simulink model "Realizacoes_Simulink_2015b"  (R2015b)
settings: Solver=ode45  SolverMode=SingleTasking  StartTime=0.0  StopTime=10.0  RelTol=1e-3
libraries: dsparch4 x4
settings Model: Creator=marco  LastModifiedBy=marco
settings DataIOCC: LimitDataPoints=off
settings DebuggingCC: AllowSymbolicDim=on  SFUnexpectedBacktrackingDiag=error  SFNoUnconditionalDefaultTransitionDiag=error
settings HardwareCC: ProdWordSize=32  ProdHWDeviceType=Specified
settings ModelReferenceCC: PropagateSignalLabelsOutOfModel=on
settings GRTTargetCC: TargetLangStandard=C99 (ISO)
settings ConfigComp: CovMetricSettings=dwe  CovHtmlReporting=off  CovSaveCumulativeToWorkspaceVar=off  CovSaveSingleToWorkspaceVar=off  CovModelRefEnable=Off  CovExternalEMLEnable=on

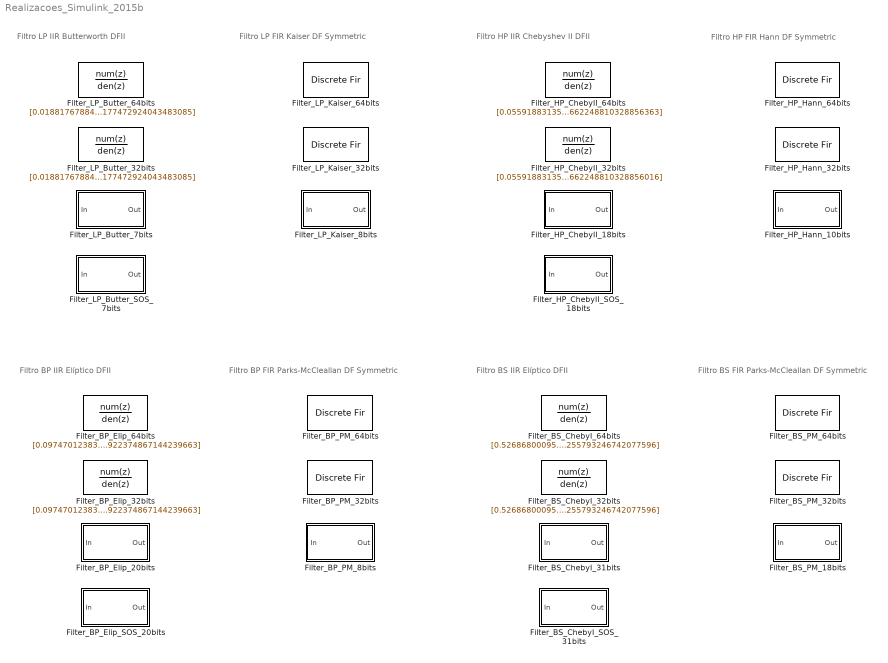
== system Realizacoes_Simulink_2015b ==
  note: Filtro LP IIR Butterworth DFII
  note: Filtro LP FIR Kaiser DF Symmetric
  note: Filtro HP IIR Chebyshev II DFII
  note: Filtro HP FIR Hann DF Symmetric
  note: Filtro BP IIR Elíptico DFII
  note: Filtro BP FIR Parks-McCleallan DF Symmetric
  note: Filtro BS IIR Elíptico DFII
  note: Filtro BS FIR Parks-McCleallan DF Symmetric
  Filter_BP_Elip_20bits : Subsystem  Tag=BlockMethodSubSystem
  Filter_BP_Elip_32bits : DiscreteFilter  Tag=BlockMethodSubSystem  Numerator=[0.0974701238336903308 0.132939383916824333 0.234899653984624923 0.132939383916824333 0.0974701238336903308]  Denominator=[1 1.35628195146766672 2.3760241493758163 1.30250572686881982 0.922374867144239663]  InputProcessing=Columns as channels (frame based)  a0EqualsOne=on
  Filter_BP_Elip_64bits : DiscreteFilter  Tag=BlockMethodSubSystem  Numerator=[0.0974701238336903308 0.132939383916824333 0.234899653984624923 0.132939383916824333 0.0974701238336903308]  Denominator=[1 1.35628195146766672 2.3760241493758163 1.30250572686881982 0.922374867144239663]  InputProcessing=Columns as channels (frame based)  a0EqualsOne=on
  Filter_BP_Elip_SOS_20bits : Subsystem  Tag=BlockMethodSubSystem
  Filter_BP_PM_32bits : DiscreteFir  Tag=BlockMethodSubSystem  FilterStructure=Direct form symmetric  Coefficients=[-0.0433412092937293658 0.00428125381265335829 0.00433549487836447974 0.00392877576103001919 0.00473672650552339151 -0.00113536747739367079 0.00225664087871407099 0.0129845358018076552 -0.00161672199950467889 -0.0104604010793571591 0.0163185558804867653 0.0128200383399435375 -0.0195811015916752505 0.00139459356195246087 0.0265908628917521095 -0.00801815848233358545 -0.0159846853288865345 0.0182879102661886624 0.00917068699111520461 -0.0101571946073742616 0.00213367932078208566 0.00146979326149086938 0.00584552068680904268 0.0142736412678231232 -0.0203435807946345457 -0.0109359709753772891 0.0481729986576425739 -0.00509592495312094235 -0.0617262707720767426 0.0445756327859687662 0.0603830661005346145 -0.0814319206649492117 -0.026284446547936522 0.110018542760450824 -0.0206200310747097909 -0.10438558333404982 0.0746608800226218894 0.0746608800226218894 -0.10438558333404982 -0.0206200310747097909 0.110018542760450824 -0.026284446547936522 -0.0814319206649492117 0.0603830661005346145 0.0445756327859687662 -0.0617262707720767426 -0.00509592495312094235 0.0481729986576425739 -0.0109359709753772891 -0.0203435807946345457 0.0142736412678231232 0.00584552068680904268 0.00146979326149086938 0.00213367932078208566 -0.0101571946073742616 0.00917068699111520461 0.0182879102661886624 -0.0159846853288865345 -0.00801815848233358545 0.0265908628917521095 0.00139459356195246087 -0.0195811015916752505 0.0128200383399435375 0.0163185558804867653 -0.0104604010793571591 -0.00161672199950467889 0.0129845358018076552 0.00225664087871407099 -0.00113536747739367079 0.00473672650552339151 0.00392877576103001919 0.00433549487836447974 0.00428125381265335829 -0.0433412092937293658]  InputProcessing=Columns as channels (frame based)
  Filter_BP_PM_64bits : DiscreteFir  Tag=BlockMethodSubSystem  FilterStructure=Direct form symmetric  Coefficients=[-0.0433412092937293658 0.00428125381265335829 0.00433549487836447974 0.00392877576103001919 0.00473672650552339151 -0.00113536747739367079 0.00225664087871407099 0.0129845358018076552 -0.00161672199950467889 -0.0104604010793571591 0.0163185558804867653 0.0128200383399435375 -0.0195811015916752505 0.00139459356195246087 0.0265908628917521095 -0.00801815848233358545 -0.0159846853288865345 0.0182879102661886624 0.00917068699111520461 -0.0101571946073742616 0.00213367932078208566 0.00146979326149086938 0.00584552068680904268 0.0142736412678231232 -0.0203435807946345457 -0.0109359709753772891 0.0481729986576425739 -0.00509592495312094235 -0.0617262707720767426 0.0445756327859687662 0.0603830661005346145 -0.0814319206649492117 -0.026284446547936522 0.110018542760450824 -0.0206200310747097909 -0.10438558333404982 0.0746608800226218894 0.0746608800226218894 -0.10438558333404982 -0.0206200310747097909 0.110018542760450824 -0.026284446547936522 -0.0814319206649492117 0.0603830661005346145 0.0445756327859687662 -0.0617262707720767426 -0.00509592495312094235 0.0481729986576425739 -0.0109359709753772891 -0.0203435807946345457 0.0142736412678231232 0.00584552068680904268 0.00146979326149086938 0.00213367932078208566 -0.0101571946073742616 0.00917068699111520461 0.0182879102661886624 -0.0159846853288865345 -0.00801815848233358545 0.0265908628917521095 0.00139459356195246087 -0.0195811015916752505 0.0128200383399435375 0.0163185558804867653 -0.0104604010793571591 -0.00161672199950467889 0.0129845358018076552 0.00225664087871407099 -0.00113536747739367079 0.00473672650552339151 0.00392877576103001919 0.00433549487836447974 0.00428125381265335829 -0.0433412092937293658]  InputProcessing=Columns as channels (frame based)
  Filter_BP_PM_8bits : Subsystem  Tag=BlockMethodSubSystem
  Filter_BS_ChebyI_31bits : Subsystem  Tag=BlockMethodSubSystem
  Filter_BS_ChebyI_32bits : DiscreteFilter  Tag=BlockMethodSubSystem  Numerator=[0.526868000951233872 -1.54203566956132732 5.62231543277647106 -10.600101182726668 21.298995446777635 -28.6634656336700679 39.4931897641130405 -39.2119772064789842 39.4931897641130405 -28.6634656336700679 21.298995446777635 -10.600101182726668 5.62231543277647106 -1.54203566956132732 0.526868000951233872]  Denominator=[1 -2.66499543662062877 8.79464618040259083 -15.0964799784515531 27.5316314023528577 -33.7583267920149481 42.2783703159670097 -38.2580281440592245 35.0287520822531278 -23.1519310706400248 15.6125822995039183 -7.05648534288835538 3.38096176201517462 -0.836935413720374832 0.255793246742077596]  InputProcessing=Columns as channels (frame based)  a0EqualsOne=on
  Filter_BS_ChebyI_64bits : DiscreteFilter  Tag=BlockMethodSubSystem  Numerator=[0.526868000951233872 -1.54203566956132732 5.62231543277647106 -10.600101182726668 21.298995446777635 -28.6634656336700679 39.4931897641130405 -39.2119772064789842 39.4931897641130405 -28.6634656336700679 21.298995446777635 -10.600101182726668 5.62231543277647106 -1.54203566956132732 0.526868000951233872]  Denominator=[1 -2.66499543662062877 8.79464618040259083 -15.0964799784515531 27.5316314023528577 -33.7583267920149481 42.2783703159670097 -38.2580281440592245 35.0287520822531278 -23.1519310706400248 15.6125822995039183 -7.05648534288835538 3.38096176201517462 -0.836935413720374832 0.255793246742077596]  InputProcessing=Columns as channels (frame based)  a0EqualsOne=on
  Filter_BS_ChebyI_SOS_31bits : Subsystem  Tag=BlockMethodSubSystem
  Filter_BS_PM_18bits : Subsystem  Tag=BlockMethodSubSystem
  Filter_BS_PM_32bits : DiscreteFir  Tag=BlockMethodSubSystem  FilterStructure=Direct form symmetric  Coefficients=[0.00939244855741547431 0.00168644324503250398 -0.00123334499269933651 0.00145794752474150894 -0.00170828863653412779 0.0010371674316927424 -0.000634686404143752943 0.00136311298569206278 -0.00129284830014917774 0.000232789421018792837 -0.000621585322147632049 0.00144095326498087451 -0.000402030343464907663 -9.93042424858531166e-05 -0.00117660388067255444 0.000857139817899975971 0.000475576697520832179 0.000566173937320908283 -0.00129976912049715575 -0.000414918760660079426 0.000263301821986200587 0.00151212084328995505 -0.000171353338375926384 -0.00112518747007188781 -0.00113282518202952216 0.00125058626817034176 0.00146260931159716097 -0.00012619100443286255 -0.00218391988276047354 -0.000599163053077525877 0.00175579742678911438 0.00189080421318403406 -0.00128579243659506307 -0.00239772150607349757 -4.34676465038889596e-05 0.0027290015939102491 0.00110819243107837312 -0.00210222575652082655 -0.00225246351867029087 0.0012254746073580233 0.00261463097525626523 0.000119119214611603793 -0.00253564082558753109 -0.00111637470738218088 0.00170231695003329351 0.0017923627508501939 -0.000727566262942802317 -0.00168402489413071446 -0.000261006656951355608 0.00111369062092454233 0.000654612245855574885 -0.000158605418687098992 -0.000457463191175657845 -0.000559561716121999351 -0.000429555092511704057 0.000760465989380783021 0.00154704577781028811 -8.44810420930140716e-05 -0.00249135328445494394 -0.00131792635448624794 0.00265371689363126401 0.00316577013999892612 -0.00178383712812358436 -0.00478209301742398528 -0.000189000463802546241 0.00558218019101575438 0.00283295693765036683 -0.00504693179469161649 -0.00550420058891909654 0.00310083210861084209 0.00739810128662848118 -3.7561071877213364e-05 -0.00788788074996699812 -0.00340775056067187066 0.00667687326885402742 0.00636929503958767306 -0.00400990072987689964 -0.00801845006079115671 0.00053623232732529229 0.00794278817684213219 0.00277147287738032603 -0.00620795501729334842 -0.00501710520110652813 0.00345225121082729913 0.00561809289207314613 -0.000643298312946369495 -0.0045743241567087296 -0.00120667662953364099 0.00248497965148512584 0.00142397294255552594 -0.000397370928880265591 5.34429434601102151e-05 -0.00054191978616790191 -0.00257813916748243126 -0.000500070247838573585 0.00493849669387566321 0.00366520397101527135 -0.00570692659790642421 -0.00825547169902910057 0.00374480093323882818 0.0128097446690955755 0.00134623112172494548 -0.0154780089784019269 -0.00894575142573483979 0.0145725727441816961 0.0174015202645732385 -0.00914885091284967263 -0.0243958071824043887 -0.000547986162959933723 0.0275080274094623607 0.012973139792518764 -0.0249501799896123012 -0.0254965656220924528 0.0161544829725067465 0.0350081953796367931 -0.00211835663899300006 -0.0387033973848105659 -0.0146670495089108472 0.0348621258612269377 0.030722101647759549 -0.023428042785332507 -0.0423658434161012024 0.00615888494345044873 0.0466417749018884706 0.0136734482850623812 -0.042103679691225207 -0.0319882017787958411 0.0292412271592478595 0.0448778449051016048 -0.0104622924834579488 0.922115113062917713 -0.0104622924834579488 0.0448778449051016048 0.0292412271592478595 -0.0319882017787958411 -0.042103679691225207 0.0136734482850623812 0.0466417749018884706 0.00615888494345044873 -0.0423658434161012024 -0.023428042785332507 0.030722101647759549 0.0348621258612269377 -0.0146670495089108472 -0.0387033973848105659 -0.00211835663899300006 0.0350081953796367931 0.0161544829725067465 -0.0254965656220924528 -0.0249501799896123012 0.012973139792518764 0.0275080274094623607 -0.000547986162959933723 -0.0243958071824043887 -0.00914885091284967263 0.0174015202645732385 0.0145725727441816961 -0.00894575142573483979 -0.0154780089784019269 0.00134623112172494548 0.0128097446690955755 0.00374480093323882818 -0.00825547169902910057 -0.00570692659790642421 0.00366520397101527135 0.00493849669387566321 -0.000500070247838573585 -0.00257813916748243126 -0.00054191978616790191 5.34429434601102151e-05 -0.000397370928880265591 ...(+2138 chars)]  InputProcessing=Columns as channels (frame based)
  Filter_BS_PM_64bits : DiscreteFir  Tag=BlockMethodSubSystem  FilterStructure=Direct form symmetric  Coefficients=[0.00939244855741547431 0.00168644324503250398 -0.00123334499269933651 0.00145794752474150894 -0.00170828863653412779 0.0010371674316927424 -0.000634686404143752943 0.00136311298569206278 -0.00129284830014917774 0.000232789421018792837 -0.000621585322147632049 0.00144095326498087451 -0.000402030343464907663 -9.93042424858531166e-05 -0.00117660388067255444 0.000857139817899975971 0.000475576697520832179 0.000566173937320908283 -0.00129976912049715575 -0.000414918760660079426 0.000263301821986200587 0.00151212084328995505 -0.000171353338375926384 -0.00112518747007188781 -0.00113282518202952216 0.00125058626817034176 0.00146260931159716097 -0.00012619100443286255 -0.00218391988276047354 -0.000599163053077525877 0.00175579742678911438 0.00189080421318403406 -0.00128579243659506307 -0.00239772150607349757 -4.34676465038889596e-05 0.0027290015939102491 0.00110819243107837312 -0.00210222575652082655 -0.00225246351867029087 0.0012254746073580233 0.00261463097525626523 0.000119119214611603793 -0.00253564082558753109 -0.00111637470738218088 0.00170231695003329351 0.0017923627508501939 -0.000727566262942802317 -0.00168402489413071446 -0.000261006656951355608 0.00111369062092454233 0.000654612245855574885 -0.000158605418687098992 -0.000457463191175657845 -0.000559561716121999351 -0.000429555092511704057 0.000760465989380783021 0.00154704577781028811 -8.44810420930140716e-05 -0.00249135328445494394 -0.00131792635448624794 0.00265371689363126401 0.00316577013999892612 -0.00178383712812358436 -0.00478209301742398528 -0.000189000463802546241 0.00558218019101575438 0.00283295693765036683 -0.00504693179469161649 -0.00550420058891909654 0.00310083210861084209 0.00739810128662848118 -3.7561071877213364e-05 -0.00788788074996699812 -0.00340775056067187066 0.00667687326885402742 0.00636929503958767306 -0.00400990072987689964 -0.00801845006079115671 0.00053623232732529229 0.00794278817684213219 0.00277147287738032603 -0.00620795501729334842 -0.00501710520110652813 0.00345225121082729913 0.00561809289207314613 -0.000643298312946369495 -0.0045743241567087296 -0.00120667662953364099 0.00248497965148512584 0.00142397294255552594 -0.000397370928880265591 5.34429434601102151e-05 -0.00054191978616790191 -0.00257813916748243126 -0.000500070247838573585 0.00493849669387566321 0.00366520397101527135 -0.00570692659790642421 -0.00825547169902910057 0.00374480093323882818 0.0128097446690955755 0.00134623112172494548 -0.0154780089784019269 -0.00894575142573483979 0.0145725727441816961 0.0174015202645732385 -0.00914885091284967263 -0.0243958071824043887 -0.000547986162959933723 0.0275080274094623607 0.012973139792518764 -0.0249501799896123012 -0.0254965656220924528 0.0161544829725067465 0.0350081953796367931 -0.00211835663899300006 -0.0387033973848105659 -0.0146670495089108472 0.0348621258612269377 0.030722101647759549 -0.023428042785332507 -0.0423658434161012024 0.00615888494345044873 0.0466417749018884706 0.0136734482850623812 -0.042103679691225207 -0.0319882017787958411 0.0292412271592478595 0.0448778449051016048 -0.0104622924834579488 0.922115113062917713 -0.0104622924834579488 0.0448778449051016048 0.0292412271592478595 -0.0319882017787958411 -0.042103679691225207 0.0136734482850623812 0.0466417749018884706 0.00615888494345044873 -0.0423658434161012024 -0.023428042785332507 0.030722101647759549 0.0348621258612269377 -0.0146670495089108472 -0.0387033973848105659 -0.00211835663899300006 0.0350081953796367931 0.0161544829725067465 -0.0254965656220924528 -0.0249501799896123012 0.012973139792518764 0.0275080274094623607 -0.000547986162959933723 -0.0243958071824043887 -0.00914885091284967263 0.0174015202645732385 0.0145725727441816961 -0.00894575142573483979 -0.0154780089784019269 0.00134623112172494548 0.0128097446690955755 0.00374480093323882818 -0.00825547169902910057 -0.00570692659790642421 0.00366520397101527135 0.00493849669387566321 -0.000500070247838573585 -0.00257813916748243126 -0.00054191978616790191 5.34429434601102151e-05 -0.000397370928880265591 ...(+2138 chars)]  InputProcessing=Columns as channels (frame based)
  Filter_HP_ChebyII_18bits : Subsystem  Tag=BlockMethodSubSystem
  Filter_HP_ChebyII_32bits : DiscreteFilter  Tag=BlockMethodSubSystem  Numerator=[0.0559188313546608654 -0.136376837541798468 0.237261208219189834 -0.275765557755878132 0.237261208219190084 -0.136376837541798718 0.0559188313546609347]  Denominator=[1 0.877081919298363322 1.20330623409765192 0.426634402615273078 0.249553249203958549 0.0208863375040826173 0.00662248810328856016]  InputProcessing=Columns as channels (frame based)  a0EqualsOne=on
  Filter_HP_ChebyII_64bits : DiscreteFilter  Tag=BlockMethodSubSystem  Numerator=[0.0559188313546608654 -0.13637683754179869 0.237261208219190139 -0.27576555775587841 0.237261208219190139 -0.13637683754179869 0.0559188313546608584]  Denominator=[1 0.877081919298363322 1.20330623409765192 0.426634402615272967 0.249553249203958494 0.0208863375040825895 0.00662248810328856363]  InputProcessing=Columns as channels (frame based)  a0EqualsOne=on
  Filter_HP_ChebyII_SOS_18bits : Subsystem  Tag=BlockMethodSubSystem
  Filter_HP_Hann_10bits : Subsystem  Tag=BlockMethodSubSystem
  Filter_HP_Hann_32bits : DiscreteFir  Tag=BlockMethodSubSystem  FilterStructure=Direct form symmetric  Coefficients=[-3.16228700308905018e-05 6.58621006149563763e-05 0.000776097424594572832 -0.00123190726621532883 -0.00166048429484726384 0.00472150775562455317 0.000207579074215400968 -0.0098865670153832335 0.00661569202063748852 0.013228130452963581 -0.0204947917682235907 -0.00852732671830981441 0.0401741168966580214 -0.0129883671048673984 -0.0612137762552903905 0.0693172305105436287 0.0774510719237060941 -0.303130389651806942 0.413280930834306504 -0.303130389651806942 0.0774510719237060941 0.0693172305105436287 -0.0612137762552903905 -0.0129883671048673984 0.0401741168966580214 -0.00852732671830981441 -0.0204947917682235907 0.013228130452963581 0.00661569202063748852 -0.0098865670153832335 0.000207579074215400968 0.00472150775562455317 -0.00166048429484726384 -0.00123190726621532883 0.000776097424594572832 6.58621006149563763e-05 -3.16228700308905018e-05]  InputProcessing=Columns as channels (frame based)
  Filter_HP_Hann_64bits : DiscreteFir  Tag=BlockMethodSubSystem  FilterStructure=Direct form symmetric  Coefficients=[-3.16228700308905018e-05 6.58621006149563763e-05 0.000776097424594572832 -0.00123190726621532883 -0.00166048429484726384 0.00472150775562455317 0.000207579074215400968 -0.0098865670153832335 0.00661569202063748852 0.013228130452963581 -0.0204947917682235907 -0.00852732671830981441 0.0401741168966580214 -0.0129883671048673984 -0.0612137762552903905 0.0693172305105436287 0.0774510719237060941 -0.303130389651806942 0.413280930834306504 -0.303130389651806942 0.0774510719237060941 0.0693172305105436287 -0.0612137762552903905 -0.0129883671048673984 0.0401741168966580214 -0.00852732671830981441 -0.0204947917682235907 0.013228130452963581 0.00661569202063748852 -0.0098865670153832335 0.000207579074215400968 0.00472150775562455317 -0.00166048429484726384 -0.00123190726621532883 0.000776097424594572832 6.58621006149563763e-05 -3.16228700308905018e-05]  InputProcessing=Columns as channels (frame based)
  Filter_LP_Butter_32bits : DiscreteFilter  Tag=BlockMethodSubSystem  Numerator=[0.0188176788491913188 0.150541430793530551 0.526895007777356872 1.05379001555471374 1.31723751944339229 1.05379001555471374 0.526895007777356872 0.150541430793530551 0.0188176788491913188]  Denominator=[1 0.169613480636834985 1.0725472360938022 0.126588905837326127 0.296672196811545885 0.0216830884738356162 0.0209853628033078755 0.000713622450830073379 0.000177472924043483085]  InputProcessing=Columns as channels (frame based)  a0EqualsOne=on
  Filter_LP_Butter_64bits : DiscreteFilter  Tag=BlockMethodSubSystem  Numerator=[0.0188176788491913188 0.150541430793530551 0.526895007777356872 1.05379001555471374 1.31723751944339229 1.05379001555471374 0.526895007777356872 0.150541430793530551 0.0188176788491913188]  Denominator=[1 0.169613480636834985 1.0725472360938022 0.126588905837326127 0.296672196811545885 0.0216830884738356162 0.0209853628033078755 0.000713622450830073379 0.000177472924043483085]  InputProcessing=Columns as channels (frame based)  a0EqualsOne=on
  Filter_LP_Butter_7bits : Subsystem  Tag=BlockMethodSubSystem
  Filter_LP_Butter_SOS_7bits : Subsystem  Tag=BlockMethodSubSystem
  Filter_LP_Kaiser_32bits : DiscreteFir  Tag=BlockMethodSubSystem  FilterStructure=Direct form symmetric  Coefficients=[0.0273632501347615166 -0.0143274016333116705 -0.0496900071545827646 0.0522341743948118928 0.0722918445052733033 -0.143149069954147889 -0.0891767371893470578 0.536803318067287871 0.961649065426961824 0.536803318067287871 -0.0891767371893470578 -0.143149069954147889 0.0722918445052733033 0.0522341743948118928 -0.0496900071545827646 -0.0143274016333116705 0.0273632501347615166]  InputProcessing=Columns as channels (frame based)
  Filter_LP_Kaiser_64bits : DiscreteFir  Tag=BlockMethodSubSystem  FilterStructure=Direct form symmetric  Coefficients=[0.0273632501347615166 -0.0143274016333116705 -0.0496900071545827646 0.0522341743948118928 0.0722918445052733033 -0.143149069954147889 -0.0891767371893470578 0.536803318067287871 0.961649065426961824 0.536803318067287871 -0.0891767371893470578 -0.143149069954147889 0.0722918445052733033 0.0522341743948118928 -0.0496900071545827646 -0.0143274016333116705 0.0273632501347615166]  InputProcessing=Columns as channels (frame based)
  Filter_LP_Kaiser_8bits : Subsystem  Tag=BlockMethodSubSystem

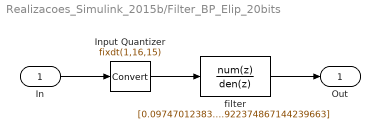
== system Realizacoes_Simulink_2015b/Filter_BP_Elip_20bits ==
  In : Inport
  Input Quantizer : DataTypeConversion  OutDataTypeStr=fixdt(1,16,15)  RndMeth=Round  SaturateOnIntegerOverflow=on
  filter : DiscreteFilter  Numerator=[0.0974701238336903308 0.132939383916824333 0.234899653984624923 0.132939383916824333 0.0974701238336903308]  Denominator=[1 1.35628195146766672 2.3760241493758163 1.30250572686881982 0.922374867144239663]  InputProcessing=Columns as channels (frame based)  a0EqualsOne=on  StateDataTypeStr=fixdt(true,16,15)  NumCoefDataTypeStr=fixdt(true,20,21)  DenCoefDataTypeStr=fixdt(true,20,17)  NumProductDataTypeStr=fixdt(true,36,36)  DenProductDataTypeStr=fixdt(true,36,32)  NumAccumDataTypeStr=fixdt(true,39,36)  DenAccumDataTypeStr=fixdt(true,39,32)  OutDataTypeStr=fixdt(true,27,24)  RndMeth=Convergent
  Out : Outport
  wires:
  In/1 -> Input Quantizer/1
  Input Quantizer/1 -> filter/1
  filter/1 -> Out/1

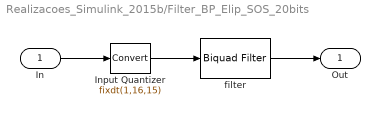
== system Realizacoes_Simulink_2015b/Filter_BP_Elip_SOS_20bits ==
  In : Inport
  Input Quantizer : DataTypeConversion  OutDataTypeStr=fixdt(1,16,15)  RndMeth=Round  SaturateOnIntegerOverflow=on
  filter : dsparch4/Biquad Filter  IIRFiltStruct=Direct form II  CoeffSource=Specify via dialog  BiQuadCoeffs=[1 0.447238317791046669 0.999999999999998002 1 0.609889161544318381 0.959873294530185661;1 0.916660471787325237 1.00000000000000311 1 0.74639278992334801 0.96093398201655611]  a0Flag=Warning  IC=0  ICnum=0  ICden=0  InputProcessing=Columns as channels (frame based)  firstCoeffMode=Binary point scaling  firstCoeffWordLength=20  firstCoeffFracLength=18  outputMode=Binary point scaling  outputWordLength=27  outputFracLength=22  accumMode=Binary point scaling  accumWordLength=38  accumFracLength=33  denAccumFracLength=33  prodOutputMode=Binary point scaling  prodOutputWordLength=36  prodOutputFracLength=33  denProdOutputFracLength=33  memoryMode=Binary point scaling  memoryWordLength=16  memoryFracLength=15  secondMemoryFracLength=15  roundingMode=Convergent  overflowMode=off  ScaleValues=[0.0974701238336903308;1;1]  optimizeScaleValues=on  ScaleValueMode=Specify via input port (g)  scaleValueFracLength=22  stageInputMode=Binary point scaling  stageOutputMode=Binary point scaling  stageInputWordLength=16  stageInputFracLength=13  stageOutputWordLength=16  stageOutputFracLength=11  FilterSource=Specify via dialog  FilterObject=BQF
  Out : Outport
  wires:
  In/1 -> Input Quantizer/1
  Input Quantizer/1 -> filter/1
  filter/1 -> Out/1

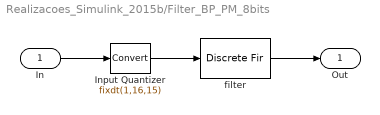
== system Realizacoes_Simulink_2015b/Filter_BP_PM_8bits ==
  In : Inport
  Input Quantizer : DataTypeConversion  OutDataTypeStr=fixdt(1,16,15)  RndMeth=Round  SaturateOnIntegerOverflow=on
  filter : DiscreteFir  FilterStructure=Direct form symmetric  Coefficients=[-0.0433412092937293658 0.00428125381265335829 0.00433549487836447974 0.00392877576103001919 0.00473672650552339151 -0.00113536747739367079 0.00225664087871407099 0.0129845358018076552 -0.00161672199950467889 -0.0104604010793571591 0.0163185558804867653 0.0128200383399435375 -0.0195811015916752505 0.00139459356195246087 0.0265908628917521095 -0.00801815848233358545 -0.0159846853288865345 0.0182879102661886624 0.00917068699111520461 -0.0101571946073742616 0.00213367932078208566 0.00146979326149086938 0.00584552068680904268 0.0142736412678231232 -0.0203435807946345457 -0.0109359709753772891 0.0481729986576425739 -0.00509592495312094235 -0.0617262707720767426 0.0445756327859687662 0.0603830661005346145 -0.0814319206649492117 -0.026284446547936522 0.110018542760450824 -0.0206200310747097909 -0.10438558333404982 0.0746608800226218894 0.0746608800226218894 -0.10438558333404982 -0.0206200310747097909 0.110018542760450824 -0.026284446547936522 -0.0814319206649492117 0.0603830661005346145 0.0445756327859687662 -0.0617262707720767426 -0.00509592495312094235 0.0481729986576425739 -0.0109359709753772891 -0.0203435807946345457 0.0142736412678231232 0.00584552068680904268 0.00146979326149086938 0.00213367932078208566 -0.0101571946073742616 0.00917068699111520461 0.0182879102661886624 -0.0159846853288865345 -0.00801815848233358545 0.0265908628917521095 0.00139459356195246087 -0.0195811015916752505 0.0128200383399435375 0.0163185558804867653 -0.0104604010793571591 -0.00161672199950467889 0.0129845358018076552 0.00225664087871407099 -0.00113536747739367079 0.00473672650552339151 0.00392877576103001919 0.00433549487836447974 0.00428125381265335829 -0.0433412092937293658]  InputProcessing=Columns as channels (frame based)  TapSumDataTypeStr=fixdt(true,17,15)  CoefDataTypeStr=fixdt(true,8,10)  ProductDataTypeStr=fixdt(true,24,25)  AccumDataTypeStr=fixdt(true,27,25)  OutDataTypeStr=fixdt(true,27,25)  RndMeth=Convergent
  Out : Outport
  wires:
  In/1 -> Input Quantizer/1
  Input Quantizer/1 -> filter/1
  filter/1 -> Out/1

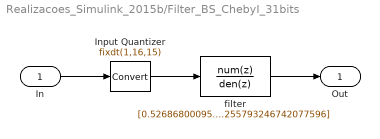
== system Realizacoes_Simulink_2015b/Filter_BS_ChebyI_31bits ==
  In : Inport
  Input Quantizer : DataTypeConversion  OutDataTypeStr=fixdt(1,16,15)  RndMeth=Round  SaturateOnIntegerOverflow=on
  filter : DiscreteFilter  Numerator=[0.526868000951233872 -1.54203566956132732 5.62231543277647106 -10.600101182726668 21.298995446777635 -28.6634656336700679 39.4931897641130405 -39.2119772064789842 39.4931897641130405 -28.6634656336700679 21.298995446777635 -10.600101182726668 5.62231543277647106 -1.54203566956132732 0.526868000951233872]  Denominator=[1 -2.66499543662062877 8.79464618040259083 -15.0964799784515531 27.5316314023528577 -33.7583267920149481 42.2783703159670097 -38.2580281440592245 35.0287520822531278 -23.1519310706400248 15.6125822995039183 -7.05648534288835538 3.38096176201517462 -0.836935413720374832 0.255793246742077596]  InputProcessing=Columns as channels (frame based)  a0EqualsOne=on  StateDataTypeStr=fixdt(true,16,15)  NumCoefDataTypeStr=fixdt(true,31,24)  DenCoefDataTypeStr=fixdt(true,31,24)  NumProductDataTypeStr=fixdt(true,47,39)  DenProductDataTypeStr=fixdt(true,47,39)  NumAccumDataTypeStr=fixdt(true,40,28)  DenAccumDataTypeStr=fixdt(true,40,28)  OutDataTypeStr=fixdt(true,16,4)  RndMeth=Convergent
  Out : Outport
  wires:
  In/1 -> Input Quantizer/1
  Input Quantizer/1 -> filter/1
  filter/1 -> Out/1

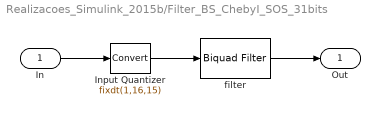
== system Realizacoes_Simulink_2015b/Filter_BS_ChebyI_SOS_31bits ==
  In : Inport
  Input Quantizer : DataTypeConversion  OutDataTypeStr=fixdt(1,16,15)  RndMeth=Round  SaturateOnIntegerOverflow=on
  filter : dsparch4/Biquad Filter  IIRFiltStruct=Direct form II  CoeffSource=Specify via dialog  BiQuadCoeffs=[1 -0.469166353343302367 1.08993846211146539 1 -0.296471121860306774 0.418147419943034726;1 -0.37804558467684346 1.08267154169078439 1 -0.0416371642925049135 0.824870003482086389;1 -0.430452143670377374 0.91748299221677887 1 -0.700389554923104618 0.837019427891170231;1 -0.349178459939221697 0.923641164997540787 1 -0.164081787063079021 0.951161413532358502;1 -0.494816477800395393 1.02358306573520808 1 -0.63968464517638346 0.953433212065612157;1 -0.321722059079580514 1.00000000285421131 1 -0.209914527018254138 0.988124396269516647;1 -0.483416033232757059 0.976960273175654259 1 -0.612816631566394543 0.988740963755510349]  a0Flag=Warning  IC=0  ICnum=0  ICden=0  InputProcessing=Columns as channels (frame based)  firstCoeffMode=Binary point scaling  firstCoeffWordLength=31  firstCoeffFracLength=29  outputMode=Binary point scaling  outputWordLength=16  outputFracLength=11  accumMode=Binary point scaling  accumWordLength=40  accumFracLength=35  denAccumFracLength=35  prodOutputMode=Binary point scaling  prodOutputWordLength=47  prodOutputFracLength=44  denProdOutputFracLength=44  memoryMode=Binary point scaling  memoryWordLength=16  memoryFracLength=15  secondMemoryFracLength=15  roundingMode=Convergent  overflowMode=off  ScaleValues=[0.526867985725402832;1;1;1;1;1;1;1]  optimizeScaleValues=on  ScaleValueMode=Specify via input port (g)  scaleValueFracLength=30  stageInputMode=Binary point scaling  stageOutputMode=Binary point scaling  stageInputWordLength=16  stageInputFracLength=10  stageOutputWordLength=16  stageOutputFracLength=11  FilterSource=Specify via dialog  FilterObject=BQF
  Out : Outport
  wires:
  In/1 -> Input Quantizer/1
  Input Quantizer/1 -> filter/1
  filter/1 -> Out/1

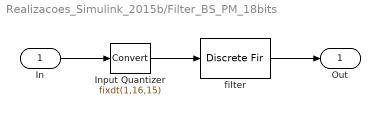
== system Realizacoes_Simulink_2015b/Filter_BS_PM_18bits ==
  In : Inport
  Input Quantizer : DataTypeConversion  OutDataTypeStr=fixdt(1,16,15)  RndMeth=Round  SaturateOnIntegerOverflow=on
  filter : DiscreteFir  FilterStructure=Direct form symmetric  Coefficients=[0.00939244855741547431 0.00168644324503250398 -0.00123334499269933651 0.00145794752474150894 -0.00170828863653412779 0.0010371674316927424 -0.000634686404143752943 0.00136311298569206278 -0.00129284830014917774 0.000232789421018792837 -0.000621585322147632049 0.00144095326498087451 -0.000402030343464907663 -9.93042424858531166e-05 -0.00117660388067255444 0.000857139817899975971 0.000475576697520832179 0.000566173937320908283 -0.00129976912049715575 -0.000414918760660079426 0.000263301821986200587 0.00151212084328995505 -0.000171353338375926384 -0.00112518747007188781 -0.00113282518202952216 0.00125058626817034176 0.00146260931159716097 -0.00012619100443286255 -0.00218391988276047354 -0.000599163053077525877 0.00175579742678911438 0.00189080421318403406 -0.00128579243659506307 -0.00239772150607349757 -4.34676465038889596e-05 0.0027290015939102491 0.00110819243107837312 -0.00210222575652082655 -0.00225246351867029087 0.0012254746073580233 0.00261463097525626523 0.000119119214611603793 -0.00253564082558753109 -0.00111637470738218088 0.00170231695003329351 0.0017923627508501939 -0.000727566262942802317 -0.00168402489413071446 -0.000261006656951355608 0.00111369062092454233 0.000654612245855574885 -0.000158605418687098992 -0.000457463191175657845 -0.000559561716121999351 -0.000429555092511704057 0.000760465989380783021 0.00154704577781028811 -8.44810420930140716e-05 -0.00249135328445494394 -0.00131792635448624794 0.00265371689363126401 0.00316577013999892612 -0.00178383712812358436 -0.00478209301742398528 -0.000189000463802546241 0.00558218019101575438 0.00283295693765036683 -0.00504693179469161649 -0.00550420058891909654 0.00310083210861084209 0.00739810128662848118 -3.7561071877213364e-05 -0.00788788074996699812 -0.00340775056067187066 0.00667687326885402742 0.00636929503958767306 -0.00400990072987689964 -0.00801845006079115671 0.00053623232732529229 0.00794278817684213219 0.00277147287738032603 -0.00620795501729334842 -0.00501710520110652813 0.00345225121082729913 0.00561809289207314613 -0.000643298312946369495 -0.0045743241567087296 -0.00120667662953364099 0.00248497965148512584 0.00142397294255552594 -0.000397370928880265591 5.34429434601102151e-05 -0.00054191978616790191 -0.00257813916748243126 -0.000500070247838573585 0.00493849669387566321 0.00366520397101527135 -0.00570692659790642421 -0.00825547169902910057 0.00374480093323882818 0.0128097446690955755 0.00134623112172494548 -0.0154780089784019269 -0.00894575142573483979 0.0145725727441816961 0.0174015202645732385 -0.00914885091284967263 -0.0243958071824043887 -0.000547986162959933723 0.0275080274094623607 0.012973139792518764 -0.0249501799896123012 -0.0254965656220924528 0.0161544829725067465 0.0350081953796367931 -0.00211835663899300006 -0.0387033973848105659 -0.0146670495089108472 0.0348621258612269377 0.030722101647759549 -0.023428042785332507 -0.0423658434161012024 0.00615888494345044873 0.0466417749018884706 0.0136734482850623812 -0.042103679691225207 -0.0319882017787958411 0.0292412271592478595 0.0448778449051016048 -0.0104622924834579488 0.922115113062917713 -0.0104622924834579488 0.0448778449051016048 0.0292412271592478595 -0.0319882017787958411 -0.042103679691225207 0.0136734482850623812 0.0466417749018884706 0.00615888494345044873 -0.0423658434161012024 -0.023428042785332507 0.030722101647759549 0.0348621258612269377 -0.0146670495089108472 -0.0387033973848105659 -0.00211835663899300006 0.0350081953796367931 0.0161544829725067465 -0.0254965656220924528 -0.0249501799896123012 0.012973139792518764 0.0275080274094623607 -0.000547986162959933723 -0.0243958071824043887 -0.00914885091284967263 0.0174015202645732385 0.0145725727441816961 -0.00894575142573483979 -0.0154780089784019269 0.00134623112172494548 0.0128097446690955755 0.00374480093323882818 -0.00825547169902910057 -0.00570692659790642421 0.00366520397101527135 0.00493849669387566321 -0.000500070247838573585 -0.00257813916748243126 -0.00054191978616790191 5.34429434601102151e-05 -0.000397370928880265591 ...(+2138 chars)]  InputProcessing=Columns as channels (frame based)  TapSumDataTypeStr=fixdt(true,17,15)  CoefDataTypeStr=fixdt(true,18,17)  ProductDataTypeStr=fixdt(true,34,32)  AccumDataTypeStr=fixdt(true,35,32)  OutDataTypeStr=fixdt(true,35,32)  RndMeth=Convergent
  Out : Outport
  wires:
  In/1 -> Input Quantizer/1
  Input Quantizer/1 -> filter/1
  filter/1 -> Out/1

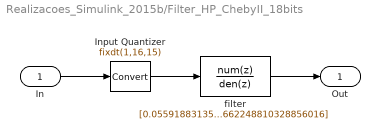
== system Realizacoes_Simulink_2015b/Filter_HP_ChebyII_18bits ==
  In : Inport
  Input Quantizer : DataTypeConversion  OutDataTypeStr=fixdt(1,16,15)  RndMeth=Round  SaturateOnIntegerOverflow=on
  filter : DiscreteFilter  Numerator=[0.0559188313546608654 -0.136376837541798468 0.237261208219189834 -0.275765557755878132 0.237261208219190084 -0.136376837541798718 0.0559188313546609347]  Denominator=[1 0.877081919298363322 1.20330623409765192 0.426634402615273078 0.249553249203958549 0.0208863375040826173 0.00662248810328856016]  InputProcessing=Columns as channels (frame based)  a0EqualsOne=on  StateDataTypeStr=fixdt(true,16,15)  NumCoefDataTypeStr=fixdt(true,18,18)  DenCoefDataTypeStr=fixdt(true,18,16)  NumProductDataTypeStr=fixdt(true,34,33)  DenProductDataTypeStr=fixdt(true,34,31)  NumAccumDataTypeStr=fixdt(true,40,33)  DenAccumDataTypeStr=fixdt(true,40,31)  OutDataTypeStr=fixdt(true,16,12)  RndMeth=Convergent
  Out : Outport
  wires:
  In/1 -> Input Quantizer/1
  Input Quantizer/1 -> filter/1
  filter/1 -> Out/1

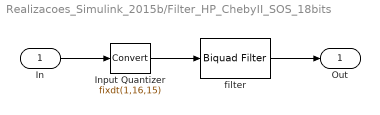
== system Realizacoes_Simulink_2015b/Filter_HP_ChebyII_SOS_18bits ==
  In : Inport
  Input Quantizer : DataTypeConversion  OutDataTypeStr=fixdt(1,16,15)  RndMeth=Round  SaturateOnIntegerOverflow=on
  filter : dsparch4/Biquad Filter  IIRFiltStruct=Direct form II  CoeffSource=Specify via dialog  BiQuadCoeffs=[1 -1.743686963462731 1.00000000000000244 1 0.0469776494469812816 0.0339719852135265121;1 -0.647343803458644285 0.999999999999998002 1 0.270775864304702851 0.278206667200348368;1 -0.0477440471859996163 1.00000000000000289 1 0.559321681560814632 0.700682609789414101]  a0Flag=Warning  IC=0  ICnum=0  ICden=0  InputProcessing=Columns as channels (frame based)  firstCoeffMode=Binary point scaling  firstCoeffWordLength=18  firstCoeffFracLength=16  outputMode=Binary point scaling  outputWordLength=16  outputFracLength=11  accumMode=Binary point scaling  accumWordLength=40  accumFracLength=31  denAccumFracLength=31  prodOutputMode=Binary point scaling  prodOutputWordLength=34  prodOutputFracLength=31  denProdOutputFracLength=31  memoryMode=Binary point scaling  memoryWordLength=16  memoryFracLength=15  secondMemoryFracLength=15  roundingMode=Convergent  overflowMode=off  ScaleValues=[0.055919647216796875;1;1;1]  optimizeScaleValues=on  ScaleValueMode=Specify via input port (g)  scaleValueFracLength=21  stageInputMode=Binary point scaling  stageOutputMode=Binary point scaling  stageInputWordLength=16  stageInputFracLength=14  stageOutputWordLength=16  stageOutputFracLength=11  FilterSource=Specify via dialog  FilterObject=BQF
  Out : Outport
  wires:
  In/1 -> Input Quantizer/1
  Input Quantizer/1 -> filter/1
  filter/1 -> Out/1

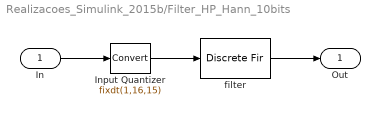
== system Realizacoes_Simulink_2015b/Filter_HP_Hann_10bits ==
  In : Inport
  Input Quantizer : DataTypeConversion  OutDataTypeStr=fixdt(1,16,15)  RndMeth=Round  SaturateOnIntegerOverflow=on
  filter : DiscreteFir  FilterStructure=Direct form symmetric  Coefficients=[-3.16228700308905018e-05 6.58621006149563763e-05 0.000776097424594572832 -0.00123190726621532883 -0.00166048429484726384 0.00472150775562455317 0.000207579074215400968 -0.0098865670153832335 0.00661569202063748852 0.013228130452963581 -0.0204947917682235907 -0.00852732671830981441 0.0401741168966580214 -0.0129883671048673984 -0.0612137762552903905 0.0693172305105436287 0.0774510719237060941 -0.303130389651806942 0.413280930834306504 -0.303130389651806942 0.0774510719237060941 0.0693172305105436287 -0.0612137762552903905 -0.0129883671048673984 0.0401741168966580214 -0.00852732671830981441 -0.0204947917682235907 0.013228130452963581 0.00661569202063748852 -0.0098865670153832335 0.000207579074215400968 0.00472150775562455317 -0.00166048429484726384 -0.00123190726621532883 0.000776097424594572832 6.58621006149563763e-05 -3.16228700308905018e-05]  InputProcessing=Columns as channels (frame based)  TapSumDataTypeStr=fixdt(true,17,15)  CoefDataTypeStr=fixdt(true,10,10)  ProductDataTypeStr=fixdt(true,26,25)  AccumDataTypeStr=fixdt(true,27,25)  OutDataTypeStr=fixdt(true,27,25)  RndMeth=Convergent
  Out : Outport
  wires:
  In/1 -> Input Quantizer/1
  Input Quantizer/1 -> filter/1
  filter/1 -> Out/1

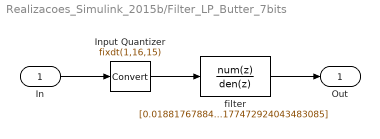
== system Realizacoes_Simulink_2015b/Filter_LP_Butter_7bits ==
  In : Inport
  Input Quantizer : DataTypeConversion  OutDataTypeStr=fixdt(1,16,15)  RndMeth=Round  SaturateOnIntegerOverflow=on
  filter : DiscreteFilter  Numerator=[0.0188176788491913188 0.150541430793530551 0.526895007777356872 1.05379001555471374 1.31723751944339229 1.05379001555471374 0.526895007777356872 0.150541430793530551 0.0188176788491913188]  Denominator=[1 0.169613480636834985 1.0725472360938022 0.126588905837326127 0.296672196811545885 0.0216830884738356162 0.0209853628033078755 0.000713622450830073379 0.000177472924043483085]  InputProcessing=Columns as channels (frame based)  a0EqualsOne=on  StateDataTypeStr=fixdt(true,16,15)  NumCoefDataTypeStr=fixdt(true,7,5)  DenCoefDataTypeStr=fixdt(true,7,5)  NumProductDataTypeStr=fixdt(true,23,20)  DenProductDataTypeStr=fixdt(true,23,20)  NumAccumDataTypeStr=fixdt(true,40,20)  DenAccumDataTypeStr=fixdt(true,40,20)  OutDataTypeStr=fixdt(true,16,9)  RndMeth=Convergent
  Out : Outport
  wires:
  In/1 -> Input Quantizer/1
  Input Quantizer/1 -> filter/1
  filter/1 -> Out/1

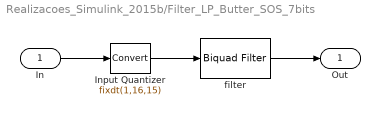
== system Realizacoes_Simulink_2015b/Filter_LP_Butter_SOS_7bits ==
  In : Inport
  Input Quantizer : DataTypeConversion  OutDataTypeStr=fixdt(1,16,15)  RndMeth=Round  SaturateOnIntegerOverflow=on
  filter : dsparch4/Biquad Filter  IIRFiltStruct=Direct form II  CoeffSource=Specify via dialog  BiQuadCoeffs=[1 1.72878589047076625 6.37424761370853243 1 0 0;1 1.99999999999999289 0.999999999999999778 1 0.357130077755224984 0.176345900779644293;1 0.271214109529229419 0.156881260440744491 1 -0.269508473259425618 0.240958472709066729;1 1.00000000000000533 0.999999999999998557 1 0.0686283955042001348 0.735431878394071092]  a0Flag=Warning  IC=0  ICnum=0  ICden=0  InputProcessing=Columns as channels (frame based)  firstCoeffMode=Binary point scaling  firstCoeffWordLength=7  firstCoeffFracLength=3  outputMode=Binary point scaling  outputWordLength=16  outputFracLength=9  accumMode=Binary point scaling  accumWordLength=40  accumFracLength=18  denAccumFracLength=20  prodOutputMode=Binary point scaling  prodOutputWordLength=23  prodOutputFracLength=18  denProdOutputFracLength=20  memoryMode=Binary point scaling  memoryWordLength=16  memoryFracLength=15  secondMemoryFracLength=15  roundingMode=Convergent  overflowMode=off  ScaleValues=[0.03125;1;1;1;1]  optimizeScaleValues=on  ScaleValueMode=Specify via input port (g)  scaleValueFracLength=10  stageInputMode=Binary point scaling  stageOutputMode=Binary point scaling  stageInputWordLength=16  stageInputFracLength=12  stageOutputWordLength=16  stageOutputFracLength=9  FilterSource=Specify via dialog  FilterObject=BQF
  Out : Outport
  wires:
  In/1 -> Input Quantizer/1
  Input Quantizer/1 -> filter/1
  filter/1 -> Out/1

== system Realizacoes_Simulink_2015b/Filter_LP_Kaiser_8bits ==
  In : Inport
  Input Quantizer : DataTypeConversion  OutDataTypeStr=fixdt(1,16,15)  RndMeth=Round  SaturateOnIntegerOverflow=on
  filter : DiscreteFir  FilterStructure=Direct form symmetric  Coefficients=[0.0273632501347615166 -0.0143274016333116705 -0.0496900071545827646 0.0522341743948118928 0.0722918445052733033 -0.143149069954147889 -0.0891767371893470578 0.536803318067287871 0.961649065426961824 0.536803318067287871 -0.0891767371893470578 -0.143149069954147889 0.0722918445052733033 0.0522341743948118928 -0.0496900071545827646 -0.0143274016333116705 0.0273632501347615166]  InputProcessing=Columns as channels (frame based)  TapSumDataTypeStr=fixdt(true,17,15)  CoefDataTypeStr=fixdt(true,8,7)  ProductDataTypeStr=fixdt(true,24,22)  AccumDataTypeStr=fixdt(true,25,22)  OutDataTypeStr=fixdt(true,25,22)  RndMeth=Convergent
  Out : Outport
  wires:
  In/1 -> Input Quantizer/1
  Input Quantizer/1 -> filter/1
  filter/1 -> Out/1
